simulink model "test_ideal_transformer"  (R2018b)
settings: Solver=VariableStepAuto  StartTime=0.0  StopTime=10.0  RelTol=1e-3
libraries: powerlib x4, typhoonHILlib x2
settings Model: Creator=USER  LastModifiedBy=USER

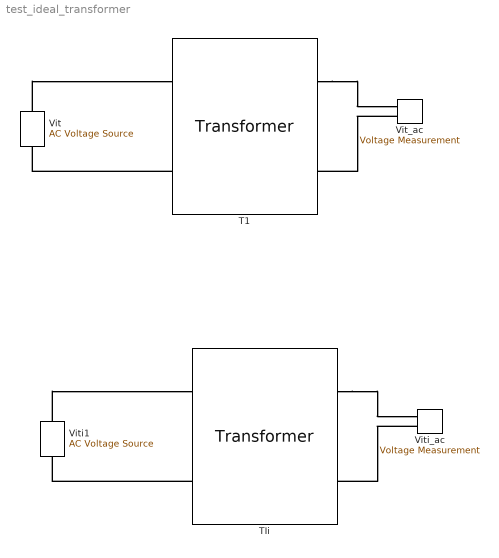
== system test_ideal_transformer ==
  T1 : typhoonHILlib/Transformer  TransfType=Single-Phase Ideal  Sn=10000  fn=50  Rm=1e5  Lm=5  sat_toggle=off  flux_vec=[0, 0.001, 0.005]  i_vec=[0, 1, 2]  n1=110  n2=220  coup12=off  coup13=off  coup14=off  units=SI  conn_1=Wye  V1=100  R1=0.1  L1=1e-3  I1=0  conn_2=Wye  V2=100  R2=0.1  L2=1e-3  I2=0  conn_3=Wye  V3=100  R3=0.1  L3=1e-3  I3=0  conn_4=Wye  V4=100  R4=0.1  L4=1e-3  I4=0  toggle_init=on  old_pat=typhoonPatterns/Ideal Transformer  old_size=145,176  model_loaded=off
      settings: SourceProductName=Typhoon HIL
  TIi : typhoonHILlib/Transformer  TransfType=Single-Phase Ideal  Sn=10000  fn=50  Rm=1e5  Lm=5  sat_toggle=off  flux_vec=[0, 0.001, 0.005]  i_vec=[0, 1, 2]  n1=110  n2=-220  coup12=off  coup13=off  coup14=off  units=SI  conn_1=Wye  V1=100  R1=0.1  L1=1e-3  I1=0  conn_2=Wye  V2=100  R2=0.1  L2=1e-3  I2=0  conn_3=Wye  V3=100  R3=0.1  L3=1e-3  I3=0  conn_4=Wye  V4=100  R4=0.1  L4=1e-3  I4=0  toggle_init=on  old_pat=typhoonPatterns/Ideal Transformer  old_size=145,176  model_loaded=off
      settings: SourceProductName=Typhoon HIL
  Vit : powerlib/Electrical Sources/AC Voltage Source  Amplitude=155.5614919  Phase=0  Frequency=50  SampleTime=0  Measurements=None  BusType=swing  Pref=10e3  Qref=0  Qmin=-inf  Qmax=+inf
  Vit_ac : powerlib/Measurements/Voltage Measurement  PhasorSimulation=off  OutputType=Complex  PSBequivalent=0
  Viti1 : powerlib/Electrical Sources/AC Voltage Source  Amplitude=155.5614919  Phase=0  Frequency=50  SampleTime=0  Measurements=None  BusType=swing  Pref=10e3  Qref=0  Qmin=-inf  Qmax=+inf
  Viti_ac : powerlib/Measurements/Voltage Measurement  PhasorSimulation=off  OutputType=Complex  PSBequivalent=0
  connections:
  Vit/RConn1 -- T1/LConn1
  T1/LConn2 -- Vit/LConn1
  T1/RConn1 -- Vit_ac/LConn1
  Vit_ac/LConn2 -- T1/RConn2
  TIi/LConn2 -- Viti1/LConn1
  TIi/RConn1 -- Viti_ac/LConn1
  Viti_ac/LConn2 -- TIi/RConn2
  Viti1/RConn1 -- TIi/LConn1
